simulink model "Simulation_Dynamics"  (R2020b)
settings: Solver=VariableStepAuto  StartTime=0.0  StopTime=10.0  RelTol=1e-3
(part 1 of 14)
settings Model: Creator=Hirsa  LastModifiedBy=Hirsa

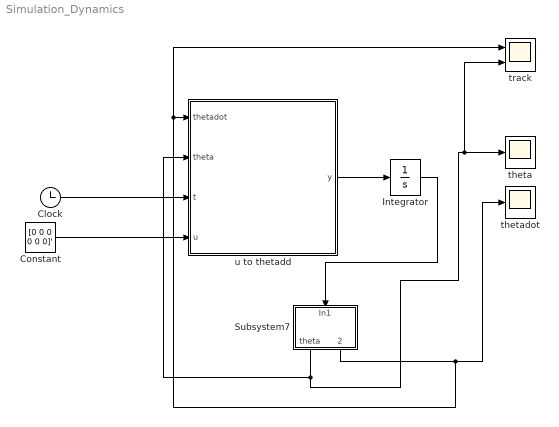
== system Simulation_Dynamics ==
  Clock : Clock
  Constant : Constant  Value=[0 0 0 0 0 0]'
  Integrator : Integrator  InitialCondition=[0.001*ones(6,1) ;zeros(6,1)]  LimitOutput=on  UpperSaturationLimit=10000  LowerSaturationLimit=-10000  AbsoluteTolerance=-1
  Subsystem7 : Subsystem
  theta : Scope
  thetadot : Scope
  track : Scope  NumInputPorts=2
  u to thetadd : MATLAB Function  TreatAsAtomicUnit=on
  wires:
  Subsystem7/2(thetadot) -> track/1, u to thetadd/1(thetadot), thetadot/1
  Subsystem7/1(theta) -> track/2, theta/1, u to thetadd/2(theta)
  Integrator/1 -> Subsystem7/1(In1)
  Clock/1 -> u to thetadd/3(t)
  u to thetadd/1(y) -> Integrator/1
  Constant/1 -> u to thetadd/4(u)

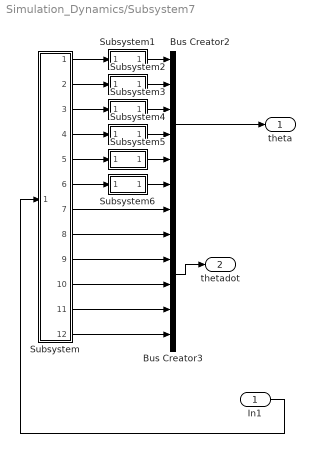
== system Simulation_Dynamics/Subsystem7 ==
  In1 : Inport
  Bus Creator2 : BusCreator  Inputs=6
  Bus Creator3 : BusCreator  Inputs=6
  Subsystem : Subsystem
  Subsystem1 : Subsystem
  Subsystem2 : Subsystem
  Subsystem3 : Subsystem
  Subsystem4 : Subsystem
  Subsystem5 : Subsystem
  Subsystem6 : Subsystem
  theta : Outport
  thetadot : Outport  Port=2
  wires:
  In1/1 -> Subsystem/1(In1)
  Subsystem/3(Out3) -> Subsystem3/1(In1)
  Subsystem/6(Out6) -> Subsystem6/1(In1)
  Subsystem/4(Out4) -> Subsystem4/1(In1)
  Subsystem/11(Out11) -> Bus Creator3/5
  Subsystem/1(Out1) -> Subsystem1/1(In1)
  Subsystem/9(Out9) -> Bus Creator3/3
  Subsystem/12(Out12) -> Bus Creator3/6
  Bus Creator2/1 -> theta/1
  Subsystem/5(Out5) -> Subsystem5/1(In1)
  Subsystem/10(Out10) -> Bus Creator3/4
  Subsystem/8(Out8) -> Bus Creator3/2
  Subsystem/2(Out2) -> Subsystem2/1(In1)
  Subsystem/7(Out7) -> Bus Creator3/1
  Bus Creator3/1 -> thetadot/1
  Subsystem2/1(Out1) -> Bus Creator2/2
  Subsystem1/1(Out1) -> Bus Creator2/1
  Subsystem6/1(Out1) -> Bus Creator2/6
  Subsystem3/1(Out1) -> Bus Creator2/3
  Subsystem4/1(Out1) -> Bus Creator2/4
  Subsystem5/1(Out1) -> Bus Creator2/5

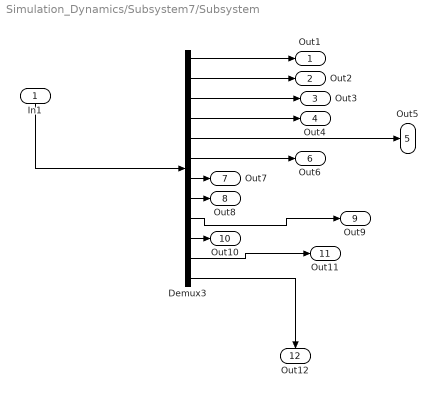
== system Simulation_Dynamics/Subsystem7/Subsystem ==
  In1 : Inport
  Demux3 : Demux  Outputs=12
  Out1 : Outport
  Out2 : Outport  Port=2
  Out3 : Outport  Port=3
  Out4 : Outport  Port=4
  Out5 : Outport  Port=5
  Out6 : Outport  Port=6
  Out7 : Outport  Port=7
  Out8 : Outport  Port=8
  Out9 : Outport  Port=9
  Out10 : Outport  Port=10
  Out11 : Outport  Port=11
  Out12 : Outport  Port=12
  wires:
  Demux3/1 -> Out1/1
  Demux3/9 -> Out9/1
  Demux3/10 -> Out10/1
  Demux3/7 -> Out7/1
  In1/1 -> Demux3/1
  Demux3/8 -> Out8/1
  Demux3/11 -> Out11/1
  Demux3/5 -> Out5/1
  Demux3/3 -> Out3/1
  Demux3/2 -> Out2/1
  Demux3/4 -> Out4/1
  Demux3/6 -> Out6/1
  Demux3/12 -> Out12/1

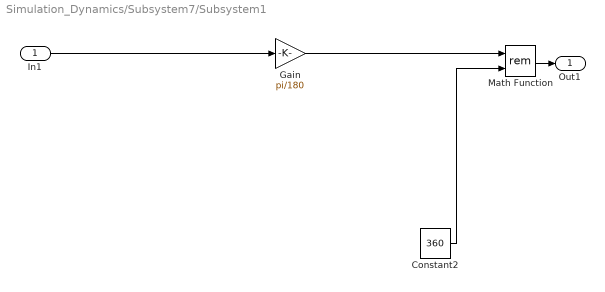
== system Simulation_Dynamics/Subsystem7/Subsystem1 ==
  In1 : Inport
  Constant2 : Constant  Value=360
  Gain : Gain  Gain=pi/180
  Math Function : Math  Operator=rem  SignedPower=on  SaturateOnIntegerOverflow=on
  Out1 : Outport
  wires:
  Math Function/1 -> Out1/1
  In1/1 -> Gain/1
  Constant2/1 -> Math Function/2
  Gain/1 -> Math Function/1

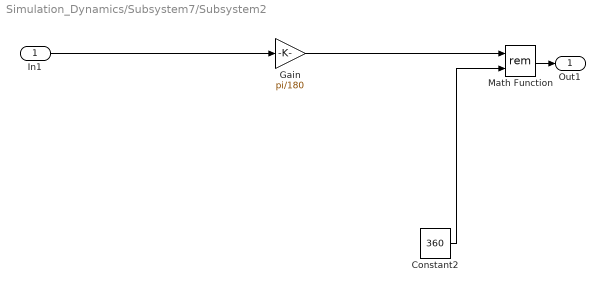
== system Simulation_Dynamics/Subsystem7/Subsystem2 ==
  In1 : Inport
  Constant2 : Constant  Value=360
  Gain : Gain  Gain=pi/180
  Math Function : Math  Operator=rem  SignedPower=on  SaturateOnIntegerOverflow=on
  Out1 : Outport
  wires:
  Math Function/1 -> Out1/1
  In1/1 -> Gain/1
  Constant2/1 -> Math Function/2
  Gain/1 -> Math Function/1

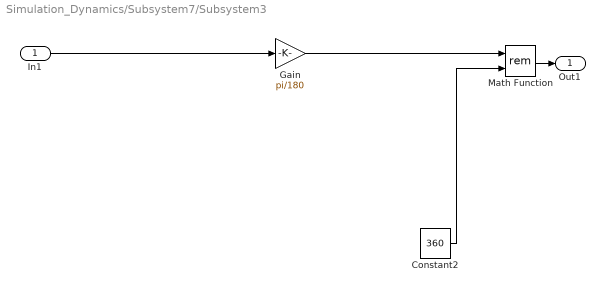
== system Simulation_Dynamics/Subsystem7/Subsystem3 ==
  In1 : Inport
  Constant2 : Constant  Value=360
  Gain : Gain  Gain=pi/180
  Math Function : Math  Operator=rem  SignedPower=on  SaturateOnIntegerOverflow=on
  Out1 : Outport
  wires:
  Math Function/1 -> Out1/1
  In1/1 -> Gain/1
  Constant2/1 -> Math Function/2
  Gain/1 -> Math Function/1

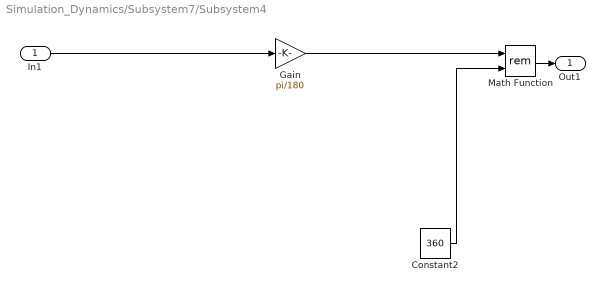
== system Simulation_Dynamics/Subsystem7/Subsystem4 ==
  In1 : Inport
  Constant2 : Constant  Value=360
  Gain : Gain  Gain=pi/180
  Math Function : Math  Operator=rem  SignedPower=on  SaturateOnIntegerOverflow=on
  Out1 : Outport
  wires:
  Math Function/1 -> Out1/1
  In1/1 -> Gain/1
  Constant2/1 -> Math Function/2
  Gain/1 -> Math Function/1

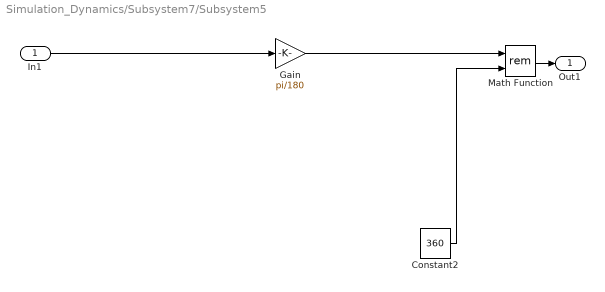
== system Simulation_Dynamics/Subsystem7/Subsystem5 ==
  In1 : Inport
  Constant2 : Constant  Value=360
  Gain : Gain  Gain=pi/180
  Math Function : Math  Operator=rem  SignedPower=on  SaturateOnIntegerOverflow=on
  Out1 : Outport
  wires:
  Math Function/1 -> Out1/1
  In1/1 -> Gain/1
  Constant2/1 -> Math Function/2
  Gain/1 -> Math Function/1

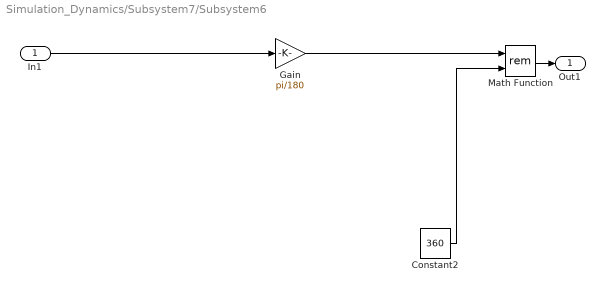
== system Simulation_Dynamics/Subsystem7/Subsystem6 ==
  In1 : Inport
  Constant2 : Constant  Value=360
  Gain : Gain  Gain=pi/180
  Math Function : Math  Operator=rem  SignedPower=on  SaturateOnIntegerOverflow=on
  Out1 : Outport
  wires:
  Math Function/1 -> Out1/1
  In1/1 -> Gain/1
  Constant2/1 -> Math Function/2
  Gain/1 -> Math Function/1
